simulink model "Block_Coding_SLX"  (R2020a)
settings: Solver=VariableStepAuto  StartTime=0.0  StopTime=5000  RelTol=1e-3
undefined symbols (not defined in the file or in its folder): dvbs2ldpc, EbNo, rsgenpoly
libraries: commsink2 x6, commblkcod2 x6, commdigbbndpm3 x6, commchan3 x3, commrandsrc3 x3
settings Model: NumberOfSteps=300  Creator=ja545  LastModifiedBy=jose_
settings SFSimCC: CustomCodeUndefinedFunction=UseInterfaceOnly

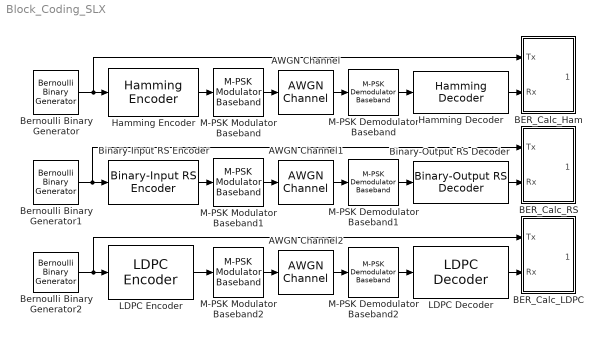
== system Block_Coding_SLX ==
  AWGN Channel : commchan3/AWGN Channel  InputProcessing=Columns as channels (frame based)  seed=67  noiseMode="Signal to noise ratio  (Eb/No)"  EbNodB=EbNo  EsNodB=10  SNRdB=10  bitsPerSym=3  Ps=1  Tsym=0.01 * 2.72  variance=1
  AWGN Channel1 : commchan3/AWGN Channel  InputProcessing=Columns as channels (frame based)  seed=67  noiseMode="Signal to noise ratio  (Eb/No)"  EbNodB=EbNo  EsNodB=10  SNRdB=10  bitsPerSym=3  Ps=1  Tsym=.52/20  variance=1
  AWGN Channel2 : commchan3/AWGN Channel  InputProcessing=Columns as channels (frame based)  seed=67  noiseMode="Signal to noise ratio  (SNR)"  EbNodB=EbNo  EsNodB=10  SNRdB=EbNo  bitsPerSym=3  Ps=1  Tsym=0.01 * 1.5  variance=1
  BER_Calc_Ham : Subsystem
  BER_Calc_LDPC : Subsystem
  BER_Calc_RS : Subsystem
  Bernoulli Binary Generator : commrandsrc3/Bernoulli Binary Generator  ProbabilityOfZero=0.5  SeedSource=Auto  Seed=0  SampleTime=0.01  SamplesPerFrame=63-6  OutputDataType=double  SimulateUsing=Interpreted execution
  Bernoulli Binary Generator1 : commrandsrc3/Bernoulli Binary Generator  ProbabilityOfZero=0.5  SeedSource=Auto  Seed=0  SampleTime=0.01  SamplesPerFrame=13*4  OutputDataType=double  SimulateUsing=Interpreted execution
  Bernoulli Binary Generator2 : commrandsrc3/Bernoulli Binary Generator  ProbabilityOfZero=0.5  SeedSource=Auto  Seed=0  SampleTime=0.01  SamplesPerFrame=32400  OutputDataType=double  SimulateUsing=Interpreted execution
  Binary-Input RS Encoder : commblkcod2/Binary-Input RS Encoder  n=15  k=13  specShortening=off  shortenedK=3  specGenPoly=off  genPoly=rsgenpoly(7, 3, [], [], 'double')  specPrimPoly=off  prPoly='X^3 + X + 1'  specPuncture=off  punctVec=[ones(2,1); zeros(2,1)]  outDType=Same as input
      settings: SourceProductBaseCode=CM
  Binary-Output RS Decoder : commblkcod2/Binary-Output RS Decoder  n=15  k=13  specShortening=off  shortenedK=3  specGenPoly=off  genPoly=rsgenpoly(7, 3, [], [], 'double')  specPrimPoly=off  prPoly='X^3 + X + 1'  specPuncture=off  punctVec=[ones(2,1); zeros(2,1)]  specErasurePort=off  showNumErr=off  outDType=Same as input
      settings: SourceProductBaseCode=CM
  Hamming Decoder : commblkcod2/Hamming Decoder  n=63  k=63-6
      settings: SourceProductBaseCode=CM
  Hamming Encoder : commblkcod2/Hamming Encoder  n=63  k=63-6
      settings: SourceProductBaseCode=CM
  LDPC Decoder : commblkcod2/LDPC Decoder  ParityCheckMat=dvbs2ldpc(1/2)  OutputFmt=Information part  DecisionType=Hard decision  OutputDataType=double  NumIter=50  DoParityCheck=off  OutputNumIter=off  OutputFinalChecks=off
      settings: SourceProductBaseCode=CM
  LDPC Encoder : commblkcod2/LDPC Encoder  ParityCheckMat=dvbs2ldpc(1/2)
      settings: SourceProductBaseCode=CM
  M-PSK Demodulator Baseband : commdigbbndpm3/M-PSK Demodulator Baseband  M=8  OutType=Bit  DecType=Hard decision  VarSource=Dialog  Variance=1  Dec=Gray  Mapping=[0:7]  Ph=0  outDtype1=Inherit via internal rule  outDtype2=Inherit via internal rule  derotateFactorWordLen=16  derotateFactorDataTypeStr=Inherit: Same word length as input  derotateFactorLastDataTypeStr=Inherit: Same word length as input
  M-PSK Demodulator Baseband1 : commdigbbndpm3/M-PSK Demodulator Baseband  M=8  OutType=Bit  DecType=Hard decision  VarSource=Dialog  Variance=1  Dec=Gray  Mapping=[0:7]  Ph=0  outDtype1=Inherit via internal rule  outDtype2=Inherit via internal rule  derotateFactorWordLen=16  derotateFactorDataTypeStr=Inherit: Same word length as input  derotateFactorLastDataTypeStr=Inherit: Same word length as input
  M-PSK Demodulator Baseband2 : commdigbbndpm3/M-PSK Demodulator Baseband  M=4  OutType=Bit  DecType=Log-likelihood ratio  VarSource=Dialog  Variance=1/db2pow(EbNo)  Dec=Gray  Mapping=[0:7]  Ph=0  outDtype1=Inherit via internal rule  outDtype2=Inherit via internal rule  derotateFactorWordLen=16  derotateFactorDataTypeStr=Inherit: Same word length as input  derotateFactorLastDataTypeStr=Inherit: Same word length as input
  M-PSK Modulator Baseband : commdigbbndpm3/M-PSK Modulator Baseband  M=8  InType=Bit  Enc=Gray  Mapping=[0:7]  Ph=0  outDtype=double  outWordLen=16  outUDDataType=sfix(16)  outFracLenMode=Best precision  outFracLen=15  outDataTypeStr=double  outLastDataTypeStr=double
  M-PSK Modulator Baseband1 : commdigbbndpm3/M-PSK Modulator Baseband  M=8  InType=Bit  Enc=Gray  Mapping=[0:7]  Ph=0  outDtype=double  outWordLen=16  outUDDataType=sfix(16)  outFracLenMode=Best precision  outFracLen=15  outDataTypeStr=double  outLastDataTypeStr=double
  M-PSK Modulator Baseband2 : commdigbbndpm3/M-PSK Modulator Baseband  M=4  InType=Bit  Enc=Gray  Mapping=[0:7]  Ph=0  outDtype=double  outWordLen=16  outUDDataType=sfix(16)  outFracLenMode=Best precision  outFracLen=15  outDataTypeStr=double  outLastDataTypeStr=double
  wires:
  M-PSK Modulator Baseband/1 -> AWGN Channel/1
  M-PSK Demodulator Baseband/1 -> Hamming Decoder/1
  Bernoulli Binary Generator/1 -> BER_Calc_Ham/1(Tx), Hamming Encoder/1
  Hamming Encoder/1 -> M-PSK Modulator Baseband/1
  Hamming Decoder/1 -> BER_Calc_Ham/2(Rx)
  AWGN Channel/1 -> M-PSK Demodulator Baseband/1
  AWGN Channel1/1 -> M-PSK Demodulator Baseband1/1
  M-PSK Demodulator Baseband1/1 -> Binary-Output RS Decoder/1
  Binary-Output RS Decoder/1 -> BER_Calc_RS/2(Rx)
  Bernoulli Binary Generator1/1 -> BER_Calc_RS/1(Tx), Binary-Input RS Encoder/1
  Binary-Input RS Encoder/1 -> M-PSK Modulator Baseband1/1
  M-PSK Modulator Baseband1/1 -> AWGN Channel1/1
  M-PSK Modulator Baseband2/1 -> AWGN Channel2/1
  LDPC Encoder/1 -> M-PSK Modulator Baseband2/1
  Bernoulli Binary Generator2/1 -> BER_Calc_LDPC/1(Tx), LDPC Encoder/1
  LDPC Decoder/1 -> BER_Calc_LDPC/2(Rx)
  M-PSK Demodulator Baseband2/1 -> LDPC Decoder/1
  AWGN Channel2/1 -> M-PSK Demodulator Baseband2/1

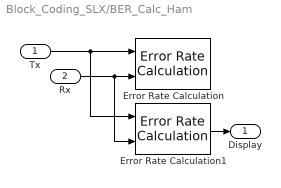
== system Block_Coding_SLX/BER_Calc_Ham ==
  Tx : Inport
  Rx : Inport  Port=2
  Error Rate Calculation : commsink2/Error Rate Calculation  N=0  st_delay=0  cp_mode=Entire frame  subframe=[]  PMode=Workspace  WsName=HammingError  RsMode2=off  stop=off  numErr=100  maxBits=1e6
  Error Rate Calculation1 : commsink2/Error Rate Calculation  N=0  st_delay=0  cp_mode=Entire frame  subframe=[]  PMode=Port  WsName=ErrorVec  RsMode2=off  stop=off  numErr=100  maxBits=1e6
  Display : Outport
  wires:
  Rx/1 -> Error Rate Calculation1/2, Error Rate Calculation/2
  Tx/1 -> Error Rate Calculation1/1, Error Rate Calculation/1
  Error Rate Calculation1/1 -> Display/1

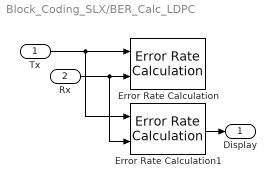
== system Block_Coding_SLX/BER_Calc_LDPC ==
  Tx : Inport
  Rx : Inport  Port=2
  Error Rate Calculation : commsink2/Error Rate Calculation  N=0  st_delay=0  cp_mode=Entire frame  subframe=[]  PMode=Workspace  WsName=LDPCError  RsMode2=off  stop=off  numErr=100  maxBits=1e6
  Error Rate Calculation1 : commsink2/Error Rate Calculation  N=0  st_delay=0  cp_mode=Entire frame  subframe=[]  PMode=Port  WsName=ErrorVec  RsMode2=off  stop=off  numErr=100  maxBits=1e6
  Display : Outport
  wires:
  Rx/1 -> Error Rate Calculation1/2, Error Rate Calculation/2
  Tx/1 -> Error Rate Calculation1/1, Error Rate Calculation/1
  Error Rate Calculation1/1 -> Display/1

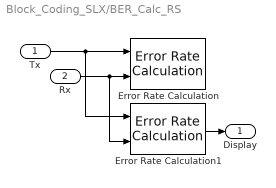
== system Block_Coding_SLX/BER_Calc_RS ==
  Tx : Inport
  Rx : Inport  Port=2
  Error Rate Calculation : commsink2/Error Rate Calculation  N=0  st_delay=0  cp_mode=Entire frame  subframe=[]  PMode=Workspace  WsName=RSError  RsMode2=off  stop=off  numErr=100  maxBits=1e6
  Error Rate Calculation1 : commsink2/Error Rate Calculation  N=0  st_delay=0  cp_mode=Entire frame  subframe=[]  PMode=Port  WsName=ErrorVec  RsMode2=off  stop=off  numErr=100  maxBits=1e6
  Display : Outport
  wires:
  Error Rate Calculation1/1 -> Display/1
  Tx/1 -> Error Rate Calculation/1, Error Rate Calculation1/1
  Rx/1 -> Error Rate Calculation/2, Error Rate Calculation1/2
